simulink model "FLOATFINALSIM"  (R2023a)
settings: Solver=VariableStepAuto  StartTime=0.0  StopTime=15  RelTol=1e-8  AbsTol=1e-8
values from neighbouring files (symbols this model uses):
  A = [0,-k/2;1/(2*m),-b/(4*m)]    [PIDF0_MATLAB.m]    (also in VelocityControl.m)
  B = [k*r/2,0; b*r/(4*m),1/m]    [PIDF0_MATLAB.m]    (also in VelocityControl.m)
  C = eye(2)    [PIDF0_MATLAB.m]    (also in VelocityControl.m)
  D = [0,0;0,0]    [PIDF0_MATLAB.m]    (also in VelocityControl.m)
  g = 9.81    [PIDF0_MATLAB.m]    (also in VelocityControl.m)
  k = 720    [PIDF0_MATLAB.m]    (also in VelocityControl.m)
  ka = .41    (= 0.41)    [PIDF0_MATLAB.m]    (also in VelocityControl.m)
  km = 0.0507    [PIDF0_MATLAB.m]    (also in VelocityControl.m)
  m = 0.5    [PIDF0_MATLAB.m]    (also in VelocityControl.m = 1)
  N = 5.9    [PIDF0_MATLAB.m]    (also in VelocityControl.m)
libraries: cstblocks x3, slpidlib x1
settings Model: Creator=Administrator  LastModifiedBy=Administrator

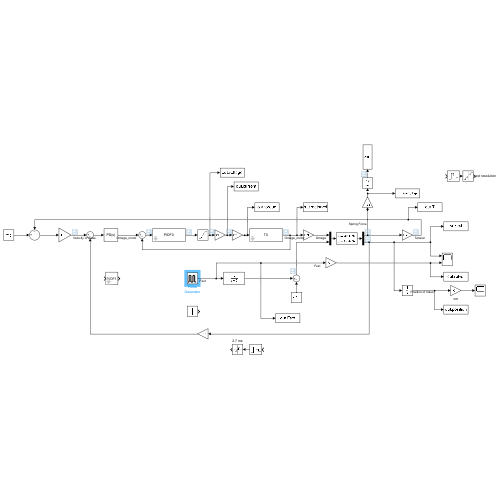
[thumbnail: Simulink's stored preview of the top-level diagram]
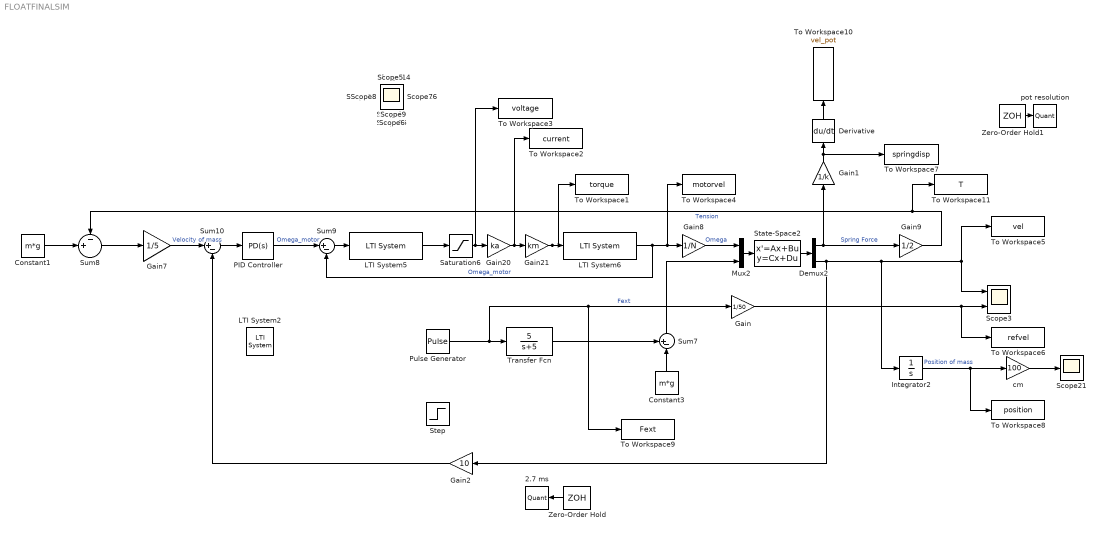
== system FLOATFINALSIM ==
  2.7 ms : Quantizer  QuantizationInterval=0.00986061724291
  Constant1 : Constant  Value=m*g  SampleTime=2.7/1000
  Constant3 : Constant  Value=m*g
  Demux2 : Demux  Outputs=2
  Derivative : Derivative
  Gain : Gain  Gain=1/50
  Gain1 : Gain  Gain=1/k
  Gain2 : Gain  Gain=10
  Gain20 : Gain  Gain=ka
  Gain21 : Gain  Gain=km
  Gain7 : Gain  Gain=1/5
  Gain8 : Gain  Gain=1/N
  Gain9 : Gain  Gain=1/2
  Integrator2 : Integrator
  LTI System2 : cstblocks/LTI System  sys=PIDF1  IC=[]
  LTI System5 : cstblocks/LTI System  sys=PIDF0  IC=[]
  LTI System6 : cstblocks/LTI System  sys=T0  IC=[]
  Mux2 : Mux  Inputs=2
  PID Controller : slpidlib/PID Controller  Controller=PD  Form=Parallel  TimeDomain=Continuous-time  UseExternalTs=off  SampleTime=-1  IntegratorMethod=Forward Euler  FilterMethod=Forward Euler  ControllerParametersSource=internal  P=544.471944741376  I=1010.02838747891  UseKiTs=off  D=8.67378620796915  N=275.981697995513  UseFilter=on  TunerSelectOption=Transfer Function Based (PID Tuner App)  InitialConditionSource=internal  InitialConditionForIntegrator=0  InitialConditionForFilter=0  DifferentiatorICPrevScaledInput=0  ExternalReset=none  TrackingMode=off  Kt=1  LimitOutput=off  SatLimitsSource=internal  UpperSaturationLimit=inf  LowerSaturationLimit=-inf  LinearizeAsGain=on  AntiWindupMode=none  Kb=1  LimitIntegrator=off  UpperIntegratorSaturationLimit=inf  LowerIntegratorSaturationLimit=-inf  POutMin=[]  POutMax=[]  IOutMin=[]  IOutMax=[]  DOutMin=[]  DOutMax=[]  NOutMin=[]  NOutMax=[]  SumOutMin=[]  SumOutMax=[]  SaturationOutMin=[]  SaturationOutMax=[]  PParamMin=[]  PParamMax=[]  IParamMin=[]  IParamMax=[]  DParamMin=[]  DParamMax=[]  NParamMin=[]  NParamMax=[]  KbParamMin=[]  KbParamMax=[]  KtParamMin=[]  KtParamMax=[]  KbOutMin=[]  KbOutMax=[]  KtOutMin=[]  KtOutMax=[]  IntegratorOutMin=[]  IntegratorOutMax=[]  FilterOutMin=[]  FilterOutMax=[]  SumI1OutMin=[]  SumI1OutMax=[]  SumI2OutMin=[]  SumI2OutMax=[]  SumI3OutMin=[]  SumI3OutMax=[]  SumI4OutMin=[]  SumI4OutMax=[]  SumDOutMin=[]  SumDOutMax=[]  DifferentiatorOutMin=[]  DifferentiatorOutMax=[]  FilterDiffOutCoefMin=[]  FilterDiffOutCoefMax=[]  ReciprocalOutMin=[]  ReciprocalOutMax=[]  SumDenOutMin=[]  SumDenOutMax=[]  SumNumOutMin=[]  SumNumOutMax=[]  DivideOutMin=[]  DivideOutMax=[]  UdiffTsProdOutMin=[]  UdiffTsProdOutMax=[]  NTsProdOutMin=[]  NTsProdOutMax=[]  UintegralTsProdOutMin=[]  UintegralTsProdOutMax=[]  UngainTsProdOutMin=[]  UngainTsProdOutMax=[]  ClampingZeroOutDataTypeStr=Inherit: Inherit via back propagation  ClampingZeroOutMin=[]  ClampingZeroOutMax=[]  FilterDenConstantOutDataTypeStr=Inherit: Inherit via back propagation  FilterDenConstantOutMin=[]  FilterDenConstantOutMax=[]  PCopyOutDataTypeStr=Inherit: Inherit via back propagation  PCopyOutMin=[]  PCopyOutMax=[]  NCopyOutDataTypeStr=Inherit: Inherit via back propagation  NCopyOutMin=[]  NCopyOutMax=[]  IntegratorContinuousStateAttributes=''  IntegratorStateMustResolveToSignalObject=off  IntegratorRTWStateStorageClass=Auto  FilterContinuousStateAttributes=''  FilterStateMustResolveToSignalObject=off  FilterRTWStateStorageClass=Auto  ParallelPVariant=InternalParameters  IdealPVariant=Disabled  IVariant=Disabled  DVariant=InternalParameters  IntegratorVariant=Disabled  SatVariant=Disabled  AWVariant=Disabled  PCopyVariant=Disabled  TRVariant=Disabled  FdbkBlocksVariant=Forward  IdealPFdbkVariant=Disabled  SatFdbkVariant=Disabled  DerivativeFilterVariant=ContFilter  NVariant=InternalParameters  NCopyVariant=Disabled  FilterICVariant=InternalICsFilter  IntegratorICVariant=Disabled  ExternalResetVariant=Disabled  TRSumVariant=Passthrough  SumFdbkVariant=Disabled  SumVariant=Sum_PD  TsampFilterVariant=InternalTs  TsampNgainVariant=Passthrough  TsampIntegralVariant=Disabled_SignalSpec  ExternalSaturationOutDataTypeStr=Inherit: Same as second input
  Pulse Generator : DiscretePulseGenerator  PulseType=Time based  Amplitude=5.8  Period=6  PulseWidth=50  PhaseDelay=3
  Saturation6 : Saturate  UpperLimit=7.5  LowerLimit=-7.5
  Scope{,1..2,4..16,21} (17 alike) : Scope
  Scope3 : Scope  NumInputPorts=2
  State-Space2 : StateSpace  A=A  B=B  C=C  D=D  InitialCondition=[2*m*g 0]
  Step : Step  Time=0  SampleTime=0
  Sum10 : Sum  Inputs=|+-
  Sum7 : Sum  Inputs=+-|
  Sum8 : Sum  Inputs=-+|
  Sum9 : Sum  Inputs=|+-
  To Workspace1 : ToWorkspace  VariableName=torque  SaveFormat=Timeseries  SampleTime=-1
  To Workspace10 : ToWorkspace  VariableName=vel_pot  SaveFormat=Timeseries  SampleTime=-1
  To Workspace11 : ToWorkspace  VariableName=T  SaveFormat=Timeseries  SampleTime=-1
  To Workspace2 : ToWorkspace  VariableName=current  SaveFormat=Timeseries  SampleTime=-1
  To Workspace3 : ToWorkspace  VariableName=voltage  SaveFormat=Timeseries  SampleTime=-1
  To Workspace4 : ToWorkspace  VariableName=motorvel  SaveFormat=Timeseries  SampleTime=-1
  To Workspace5 : ToWorkspace  VariableName=vel  SaveFormat=Timeseries  SampleTime=-1
  To Workspace6 : ToWorkspace  VariableName=refvel  SaveFormat=Timeseries  SampleTime=-1
  To Workspace7 : ToWorkspace  VariableName=springdisp  SaveFormat=Timeseries  SampleTime=-1
  To Workspace8 : ToWorkspace  VariableName=position  SaveFormat=Timeseries  SampleTime=-1
  To Workspace9 : ToWorkspace  VariableName=Fext  SaveFormat=Timeseries  SampleTime=-1
  Transfer Fcn : TransferFcn  Numerator=[5]  Denominator=[1 5]
  Zero-Order Hold : ZeroOrderHold  SampleTime=2.7/1000
  Zero-Order Hold1 : ZeroOrderHold  SampleTime=2.7/1000
  cm : Gain  Gain=100
  pot resolution : Quantizer  QuantizationInterval=0.0126
  wires:
  Pulse Generator/1 -> To Workspace9/1, Gain/1, Transfer Fcn/1  "Fext"
  LTI System6/1 -> To Workspace4/1, Gain8/1, Sum9/2  "Omega_motor"
  Constant3/1 -> Sum7/2
  Sum9/1 -> LTI System5/1
  Gain7/1 -> Sum10/1  "Velocity of mass"
  Gain20/1 -> To Workspace2/1, Gain21/1
  Gain9/1 -> To Workspace11/1, Sum8/1  "Tension"
  Gain21/1 -> To Workspace1/1, LTI System6/1
  Mux2/1 -> State-Space2/1
  Gain/1 -> To Workspace6/1, Scope3/2
  Gain8/1 -> Mux2/1  "Omega"
  Integrator2/1 -> To Workspace8/1, cm/1  "Position of mass"
  Sum7/1 -> Mux2/2
  Sum8/1 -> Gain7/1
  Demux2/1 -> Gain9/1, Gain1/1  "Spring Force"
  PID Controller/1 -> Sum9/1  "Omega_motor"
  Transfer Fcn/1 -> Sum7/1
  cm/1 -> Scope21/1
  Gain1/1 -> Derivative/1, To Workspace7/1
  Derivative/1 -> To Workspace10/1
  State-Space2/1 -> Demux2/1
  LTI System5/1 -> Saturation6/1
  Saturation6/1 -> To Workspace3/1, Gain20/1
  Zero-Order Hold/1 -> 2.7 ms/1
  Zero-Order Hold1/1 -> pot resolution/1
  Demux2/2 -> Gain2/1, To Workspace5/1, Scope3/1, Integrator2/1
  Constant1/1 -> Sum8/2
  Sum10/1 -> PID Controller/1
  Gain2/1 -> Sum10/2
